simulink library "allocation_logic"  (R2018b)
settings: Solver=VariableStepAuto  StartTime=0.0  StopTime=10.0  RelTol=1e-3
undefined symbols (not defined in the file): fswParams
settings Model: Creator=colem  LastModifiedBy=colem

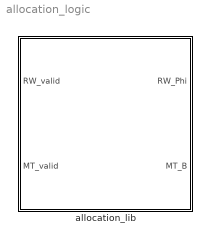
== system allocation_logic ==
  allocation_lib : Subsystem

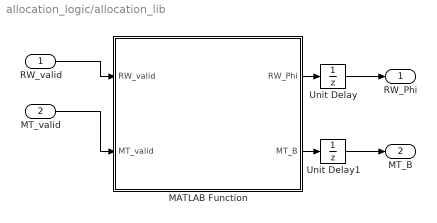
== system allocation_logic/allocation_lib ==
  RW_valid : Inport
  MT_valid : Inport  Port=2
  MATLAB Function : MATLAB Function  TreatAsAtomicUnit=on
  Unit Delay : UnitDelay  InitialCondition=fswParams.allocator.Phi  SampleTime=-1
  Unit Delay1 : UnitDelay  InitialCondition=[1 1 1 1 1]  SampleTime=-1
  RW_Phi : Outport
  MT_B : Outport  Port=2
  wires:
  Unit Delay/1 -> RW_Phi/1
  RW_valid/1 -> MATLAB Function/1(RW_valid)
  MATLAB Function/1(RW_Phi) -> Unit Delay/1
  MT_valid/1 -> MATLAB Function/2(MT_valid)
  MATLAB Function/2(MT_B) -> Unit Delay1/1
  Unit Delay1/1 -> MT_B/1

== matlab function allocation_logic/allocation_lib/MATLAB Function ==
  data: RW_valid input; RW_Phi output; MT_valid input; MT_B output
% Logic for selecting the gnc allocation scheme
%
% Author: Cole Morgan 
%
% 



function [RW_Phi, MT_B]  = allocation_logic(RW_valid, MT_valid)

%GNC_ALLOCATION_LOGIC    GNC Allocation Selector
%
% Chooses allocation scheme based on actuator validity.
%   RW_Phi = The mapping from u_c (the 3x1 total body-frame torque command)
%       to tau_c (the 4x1 vector of comanded torques to each individual wheel).
%       This is a 4x3 mapping. 4 wheels, distrubuted over 3 directions.
%   MT_B = A vector containing the necessary gain to each MT. Recall, the MTs are
%       alligned with the body axes. Therefore a torque commanded in the
%       body frame passes "straight through", only to be gained depending
%       on availability or direction. The notation is: [+x -x +y -y +z].
%       An example is [1 -1 0 -1 1] indicating that the +y-face MT is
%       unoperational.
%
% ----- INPUTS -----
%
% 1. RW_valid - a 1x4 vector containing the availability of the 4 RWA wheels.
%       An example is [1 1 0 1], which indicates that wheel_3 is
%       unoperational. The RW_Phi mapping changes accordingly.
%
% 2. MT_valid - a 1x5 vector containing the availability of the 5 Magnetorquers.
%       An example is [1 1 0 1 1], which indicates that +y-face MT is
%       unoperational. The MT_B mapping (gain) changes accordingly.
%
% -------------------------------------------------------------------------------



% Assume all actuators are availabe.
RW_Phi     = fswParams.allocator.Phi;
MT_B       = [1 -1 1 -1 1];

%check how many RWA wheels are dead
num_dead = sum(RW_valid == 0);

if (num_dead > 0 && num_dead < 2)
    
    % zeros the column of dead wheel from A
    temp = fswParams.allocator.A*diag([RW_valid]);
    RW_Phi = temp'/(temp*temp');
    % This method does not work if two wheels are dead
    % becuase two vectors cannot span R3. Then RW_Phi
    % will be NaN. inv of singular matrix.
    
%     if (RW_valid == [0 1 1 1])
%         RW_Phi = fswParams.allocator.Phi_1;
%     elseif (RW_valid == [1 0 1 1])
%         RW_Phi = fswParams.allocator.Phi_2;
%     elseif (RW_valid == [1 1 0 1])
%         RW_Phi = fswParams.allocator.Phi_3;
%     elseif (RW_valid == [1 1 1 0])
%         RW_Phi = fswParams.allocator.Phi_4;
%     end
% end
% % notice that if two wheels are dead, the default Phi will still
% % be used. This is a potential problem.

elseif(num_dead >= 2)
    
    % Uses the original Phi but zeros the dead columns of Phi.
    % note this will not be an optimal Phi, but it seems better than
    % doing nothing.
    RW_Phi = diag([RW_valid])*RW_Phi;
end

% check if any MTs are dead
if (MT_valid != [1 1 1 1 1])
    
    MT_B = MT_valid.*MT_B;
    
%     if (MT_valid == [0 1 1 1 1])
%         MT_B = [0 -2 1 1 1];
%     elseif (MT_valid == [1 0 1 1 1])
%         MT_B = [2 0 1 1 1];
%     elseif (MT_valid == [1 1 0 1 1])
%         MT_B = [1 -1 0 -2 1];
%     elseif (MT_valid == [1 1 1 0 1])
%         MT_B = [1 -1 2 0 1];
%     elseif (MT_valid == [1 1 1 1 0])
%         MT_B = [1 -1 1 -1 0];
%     end
% % notice that if two MTs are dead, the default gain will still
% % be used. This is a potential problem.
    
end
